simulink model "ilc_ramp"  (Simulink 8.7)
settings: Solver=ode45  StartTime=0.0  StopTime=2000  RelTol=1e-3
libraries: simulink x1
settings Model: Creator=aeagr  LastModifiedBy=aeagr
settings DataIOCC: SignalLoggingSaveFormat=ModelDataLogs
settings OptimizationCC: ExpressionDepthLimit=2147483647
settings DebuggingCC: SolverPrmCheckMsg=warning  FcnCallInpInsideContextMsg=EnableAllAsWarning  StateNameClashWarn=warning

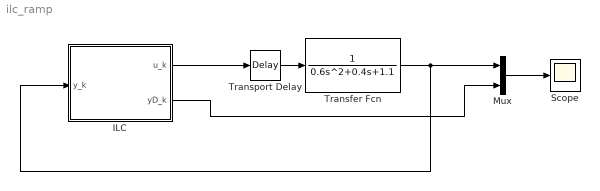
== system ilc_ramp ==
  ILC : Subsystem  Description=Iterative Learning Control  TreatAsAtomicUnit=on  SystemSampleTime=dt  mask{Yseq=[zeros(1,30) 1:30 30*ones(1,30) 29:-1:0]/30, dt=1, gamma=0.2}
      mask prompts: Yseq "Target output sequence"; dt "Time step"; gamma "Learning rate"
  Mux : Mux  Inputs=2
  Scope : Scope
  Transfer Fcn : TransferFcn  Denominator=[0.6 0.4 1.1]
  Transport Delay : TransportDelay  DelayTime=0.3
  wires:
  Transfer Fcn/1 -> ILC/1(y_k), Mux/1
  Mux/1 -> Scope/1
  ILC/2(yD_k) -> Mux/2
  ILC/1(u_k) -> Transport Delay/1
  Transport Delay/1 -> Transfer Fcn/1

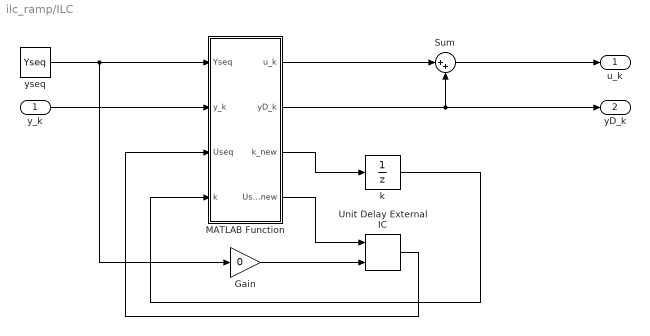
== system ilc_ramp/ILC ==
  y_k : Inport
  Gain : Gain  Gain=0
  MATLAB Function : MATLAB Function  TreatAsAtomicUnit=on
  Sum : Sum  Inputs=|++
  Unit Delay External IC : simulink/Additional Math & Discrete/Additional Discrete/Unit Delay External IC  tsamp=-1
  k : UnitDelay  InitialCondition=1  SampleTime=-1
  yseq : Constant  Value=Yseq
  u_k : Outport
  yD_k : Outport  Port=2
  wires:
  MATLAB Function/3(k_new) -> k/1
  MATLAB Function/4(Useq_new) -> Unit Delay External IC/1
  Unit Delay External IC/1 -> MATLAB Function/3(Useq)
  y_k/1 -> MATLAB Function/2(y_k)
  yseq/1 -> MATLAB Function/1(Yseq), Gain/1
  k/1 -> MATLAB Function/4(k)
  MATLAB Function/2(yD_k) -> Sum/2, yD_k/1
  Sum/1 -> u_k/1
  MATLAB Function/1(u_k) -> Sum/1
  Gain/1 -> Unit Delay External IC/2

== matlab function ILC/MATLAB Function ==
  data: u_k output double; Yseq input double; yD_k output double; y_k input double; Useq input double; k input double; k_new output double; Useq_new output double; gamma parameter double
function [u_k,yD_k,k_new,Useq_new] = fcn(Yseq,y_k,Useq,k,gamma)
%#codegen

% number of elements in sequence
Nseq = numel(Yseq);

% counter
k_new = k+1;
% reset if we've been round the sequence
if k_new>Nseq,
    k_new=1;
end

% extract current demand signal
yD_k = Yseq(k);

% and the current control
u_k = Useq(k);

% form the error
e_k = yD_k - y_k;

% copy the control sequence over
Useq_new = Useq;

% which entry to update
k_learn = k-1;
if k_learn<1,
    k_learn=Nseq;
end

% do the learning update
Useq_new(k_learn) = Useq_new(k_learn) + gamma*e_k;
